simulink model "planmodel2023b"  (R2023b)
settings: Solver=ode4  StartTime=0.0  StopTime=50  FixedStep=0.001  RelTol=1e-3
values from neighbouring files (symbols this model uses):
  a0 = 340.294    [basedata.m]    (also in basedata.mat; control_design.mat; landing_init.m; landing_plan.mat)
  b_ref = 2.0    (= 2)    [basedata.m]    (also in basedata.mat; control_design.mat; landing_init.m; landing_plan.mat)
  c_gear = [0.8e4, 1.4e4, 1.4e4]    [basedata.m]    (also in basedata.mat = [8000 14000 14000]; control_design.mat = [8000 14000 14000]; landing_init.m; landing_plan.mat = [8000 14000 14000])
  c_lat = [1.4e4, 2.2e4, 2.2e4]    [basedata.m]    (also in basedata.mat = [14000 22000 22000]; control_design.mat = [14000 22000 22000]; landing_init.m; landing_plan.mat = [14000 22000 22000])
  c_ref = 0.9    [basedata.m]    (also in basedata.mat; control_design.mat; landing_init.m; landing_plan.mat)
  c_roll = [0.020, 0.018, 0.018]    [basedata.m]    (also in basedata.mat = [0.02 0.018 0.018]; control_design.mat = [0.02 0.018 0.018]; landing_init.m; landing_plan.mat = [0.02 0.018 0.018])
  CD0 = 0.045    [basedata.m]    (also in basedata.mat; canshujisuan.m; control_design.mat; landing_init.m)
  CL0 = 0.083    [basedata.m]    (also in basedata.mat; control_design.mat; landing_init.m; landing_plan.mat)
  CLa = 3.80    (= 3.8)    [basedata.m]    (also in basedata.mat; canshujisuan.m = 2.5; control_design.mat; landing_init.m)
  Clb = -0.08    [basedata.m]    (also in basedata.mat; control_design.mat; landing_init.m; landing_plan.mat)
  Clda = -0.20    (= -0.2)    [basedata.m]    (also in basedata.mat; control_design.mat; landing_init.m; landing_plan.mat)
  CLde = 0.28    [basedata.m]    (also in basedata.mat; control_design.mat; landing_init.m; landing_plan.mat)
  Clp = -0.70    (= -0.7)    [basedata.m]    (also in basedata.mat; control_design.mat; landing_init.m; landing_plan.mat)
  CLq = 4.50    (= 4.5)    [basedata.m]    (also in basedata.mat; canshujisuan.m = 3; control_design.mat; landing_init.m)
  Clr = 0.08    [basedata.m]    (also in basedata.mat; control_design.mat; landing_init.m; landing_plan.mat)
  Cm0 = 0.060    (= 0.06)    [basedata.m]    (also in basedata.mat; control_design.mat; landing_init.m; landing_plan.mat)
  Cma = -0.80    (= -0.8)    [basedata.m]    (also in basedata.mat; control_design.mat; landing_init.m; landing_plan.mat)
  Cmde = -0.90    (= -0.9)    [basedata.m]    (also in basedata.mat; control_design.mat; landing_init.m; landing_plan.mat)
  Cmq = -18.0    (= -18)    [basedata.m]    (also in basedata.mat; control_design.mat; landing_init.m; landing_plan.mat)
  Cnb = 0.25    [basedata.m]    (also in basedata.mat; control_design.mat; landing_init.m; landing_plan.mat)
  Cndr = -0.15    [basedata.m]    (also in basedata.mat; control_design.mat; landing_init.m; landing_plan.mat)
  Cnp = -0.04    [basedata.m]    (also in basedata.mat; control_design.mat; landing_init.m; landing_plan.mat)
  Cnr = -0.45    [basedata.m]    (also in basedata.mat; control_design.mat; landing_init.m; landing_plan.mat)
  CSb = -0.70    (= -0.7)    [basedata.m]    (also in basedata.mat; control_design.mat; landing_init.m; landing_plan.mat)
  CSdr = 0.18    [basedata.m]    (also in basedata.mat; control_design.mat; landing_init.m; landing_plan.mat)
  CSr = 0.12    [basedata.m]    (also in basedata.mat; control_design.mat; landing_init.m; landing_plan.mat)
  D = 0.5 * rho0 * V^2 * S_ref * CD_current    [canshujisuan.m]
  D0 = 1400    [basedata.m]    (also in basedata.mat; control_design.mat = 800; landing.m; landing_init.m)
  da_max = 25    [basedata.m]    (also in basedata.mat; control_design.mat; landing_init.m; landing_plan.mat)
  da_min = -da_max    (= -25)    [basedata.m]    (also in basedata.mat; control_design.mat; landing_init.m; landing_plan.mat)
  de_max = 25    [basedata.m]    (also in basedata.mat; control_design.mat; landing_init.m; landing_plan.mat)
  de_min = -de_max    (= -25)    [basedata.m]    (also in basedata.mat; control_design.mat; landing_init.m; landing_plan.mat)
  DH = pi / 180    (= 0.0174532925199)    [basedata.m]    (also in basedata.mat; control_design.mat; landing_init.m; landing_plan.mat)
  dr_max = 25    [basedata.m]    (also in basedata.mat; control_design.mat; landing_init.m; landing_plan.mat)
  dr_min = -dr_max    (= -25)    [basedata.m]    (also in basedata.mat; control_design.mat; landing_init.m; landing_plan.mat)
  g = 9.80665    [basedata.m]    (also in basedata.mat; canshujisuan.m; control_design.mat; landing_init.m)
  gamma0 = 0.0    (= 0)    [plan.m]    (also in plan.mat)
  ground_y = 0.0    (= 0)    [plan.m]    (also in plan.mat)
  HD = 180 / pi    (= 57.2957795131)    [basedata.m]    (also in basedata.mat; control_design.mat; landing_init.m; landing_plan.mat)
  Ixx = 120.0    (= 120)    [basedata.m]    (also in basedata.mat; control_design.mat; landing_init.m; landing_plan.mat)
  Iyy = 480.0    (= 480)    [basedata.m]    (also in basedata.mat; control_design.mat; landing_init.m; landing_plan.mat)
  Izz = 520.0    (= 520)    [basedata.m]    (also in basedata.mat; control_design.mat; landing_init.m; landing_plan.mat)
  K = 0.12    [basedata.m]    (also in basedata.mat; canshujisuan.m = 0.08; control_design.mat; landing_init.m)
  K_alpha = 7.5375    [basedata.mat]    (also in control_design.m = (((wd_pitch^2)-a24))/(2*kesi_pitch*wd_pitch); control_design.mat; controller.m = 9.375; landingplan.mat)
  k_gear = [1.0e5, 3.0e5, 3.0e5]    [basedata.m]    (also in basedata.mat = [100000 300000 300000]; control_design.mat = [100000 300000 300000]; landing_init.m; landing_plan.mat = [100000 300000 300000])
  k_theta0 = 0.0    (= 0)    [plan.m]    (also in plan.mat)
  Kn_pitch = -0.120095403309    [basedata.mat]    (also in control_design.m = -(2.2*g*(wd_pitch)^2)/(Tr*(((wd_pitch)^2)-a24)*V_control*a34; control_design.mat; controller.m = (2.2*wd^2*g)/(Tr*(wd^2-a24)*V_test*a34); landingplan.mat)
  Kw_pitch = -0.483749055178    [basedata.mat]    (also in control_design.m = -2*kesi_pitch*wd_pitch/a25; control_design.mat; controller.m = -(2*zeta*wd) / a25; landingplan.mat)
  m = 600.0    (= 600)    [basedata.m]    (also in basedata.mat; canshujisuan.m; control_design.mat; landing_init.m)
  mu_brake = [0.0, 0.55, 0.55]    [basedata.m]    (also in basedata.mat = [0 0.55 0.55]; control_design.mat = [0 0.55 0.55]; landing_init.m; landing_plan.mat = [0 0.55 0.55])
  omigax0 = 0    [plan.m]    (also in plan.mat)
  omigay0 = 0    [plan.m]    (also in plan.mat)
  omigaz0 = 0    [plan.m]    (also in plan.mat)
  psi0 = 0    [control_design.mat]    (also in landing.m; landing_init.m; landing_init.mat; landing_plan.mat)
  r_left_b = r_gear_b(:,2)    [basedata.m]    (also in basedata.mat = [-0.333333333333 -0.8 0.65]; control_design.mat = [-0.333333333333 -0.8 0.65]; landing_init.m; landing_plan.mat = [-0.333333333333 -0.8 0.65])
  r_nose_b = r_gear_b(:,1)    [basedata.m]    (also in basedata.mat = [2 0 0.65]; control_design.mat = [2 0 0.65]; landing_init.m; landing_plan.mat = [2 0 0.65])
  r_right_b = r_gear_b(:,3)    [basedata.m]    (also in basedata.mat = [-0.333333333333 0.8 0.65]; control_design.mat = [-0.333333333333 0.8 0.65]; landing_init.m; landing_plan.mat = [-0.333333333333 0.8 0.65])
  rho0 = 1.225    [basedata.m]    (also in basedata.mat; canshujisuan.m; control_design.mat; landing_init.m)
  S_ref = 1.2    [basedata.m]    (also in basedata.mat; canshujisuan.m; control_design.mat; landing_init.m)
  v_eps = 0.20    (= 0.2)    [basedata.m]    (also in basedata.mat; control_design.mat; landing_init.m; landing_plan.mat)
  V_min = 3    [control_design.mat]    (also in landing.m; landing_init.m; landing_plan.mat; landingplan.mat)
  Vx0_b = 0.0    (= 0)    [plan.m]    (also in plan.mat)
  Vy0_b = 0.0    (= 0)    [plan.m]    (also in plan.mat)
  Vz0_b = 0.0    (= 0)    [plan.m]    (also in plan.mat)
  wheel_radius = 0.18    [basedata.m]    (also in basedata.mat; control_design.mat; landing_init.m; landing_plan.mat)
  WOW_on = 0.000    (= 0)    [basedata.m]    (also in basedata.mat; control_design.mat; landing_init.m; landing_plan.mat)
  Xg0 = 0    [control_design.mat]    (also in landing.m = -12000; landing_init.m = -12000; landing_init.mat = -8000; landing_plan.mat = -12000)
  Yg0 = 3    [control_design.mat]    (also in landing.m = 0; landing_init.m = 0; landing_init.mat = 0; landing_plan.mat = 0)
  Zg0 = ground_z - wheel_radius - r_gear_b(3,1) + static_deflection    [basedata.m]    (also in basedata.mat = -0.8215943; control_design.mat = -0.8215943; landing.m = -1000; landing_init.m = -1000)
libraries: matrix_library x18, slpidlib x1
(part 3 of 3)

== matlab function planmodel2023b/control/MATLAB Function ==
  settings: updateMethod=DISCRETE
  data: Vx input; theta_cmd output; no_contact input; t input; theta_actual input
function theta_cmd = fcn(Vx, no_contact, t, theta_actual)
% 起飞抬前轮俯仰角指令生成
% Vx:           机体系前向速度 (m/s)
% no_contact:   无轮接地信号, 1=空中, 0=地面
% t:            仿真时间 (s), 接 Digital Clock
% theta_actual: 飞机当前的实际俯仰角 (rad), 用于离地无缝切换

persistent t_rotation
persistent theta_takeoff_hold

if isempty(t_rotation)
    t_rotation = inf;
end
if isempty(theta_takeoff_hold)
    theta_takeoff_hold = 0;
end

%% --- 参数配置（根据实际机型调整） ---
VR = 50;                      % m/s, 抬轮速度 
theta_target = 12 * pi/180;   % rad, 目标俯仰角锁定在 10°
rotation_rate = 4 * pi/180;   % rad/s, 抬轮角速率设定为 3°/s，平稳抬头

%% --- 状态机控制逻辑 ---
if no_contact > 0.5
    % 【空中阶段】
    % 刚离地瞬间，记录下离地时的实际姿态，防止指令断崖式下掉
    if theta_takeoff_hold == 0
        theta_takeoff_hold = theta_actual; 
    end
    
    % 在这里，theta_cmd 应该输出离地锁定的姿态，或者直接交给空中的俯仰回路
    % 绝对不能直接置 0！
    theta_cmd = theta_takeoff_hold; 
    
    % 重置滑跑计时器
    t_rotation = inf;

elseif Vx >= VR
    % 【抬轮阶段】
    if isinf(t_rotation)
        t_rotation = t;       % 记录开始抬轮的绝对时间
    end
    
    % 按照设定的速率（3°/s）线性增加俯仰角指令
    theta_cmd = rotation_rate * (t - t_rotation);
    
    % 达到目标角度（10°）后进行限幅切顶
    if theta_cmd > theta_target
        theta_cmd = theta_target;
    end
    
    % 尚未离地，清空离地保持值
    theta_takeoff_hold = 0;

else
    % 【地面加速滑跑阶段】
    % 保持前轮三点接地姿态（通常为 0° 或略微带一点下俯角压前轮，视安装角而定）
    theta_cmd = -4*pi/180; 
    t_rotation = inf;
    theta_takeoff_hold = 0;
end% 在你的状态机逻辑中添加：

end

== matlab function planmodel2023b/6DOF-MODEL/动力学/体系旋转角速度/MATLAB Function ==
  data: alpha input; R_wind_b output; beta input
 function R_wind_b = wind2body(alpha, beta)
T1 = [cos(beta), 0, -sin(beta);
       0, 1, 0;
       sin(beta), 0, cos(beta)];
T2 = [cos(alpha), sin(alpha), 0;
       -sin(alpha), cos(alpha), 0;
       0, 0, 1];
R_wind_b = T2*T1;

== matlab function planmodel2023b/6DOF-MODEL/动力学/Subsystem3/MATLAB Function1 ==
  data: gamma input; R_gb output; theta input; psi input
function R_gb = ground2body(gamma, theta, psi)
    T1=[cos(psi), 0 ,-sin(psi);...
          0     , 1 ,    0   ;...
        sin(psi), 0 ,cos(psi);];%绕y偏航
    T2=[cos(theta),sin(theta),0;...
        -sin(theta),cos(theta),0;...
          0        , 0 ,       1;];%绕z俯仰角
    T3=[1,0,0;...
        0,cos(gamma),sin(gamma);...
        0,-sin(gamma),cos(gamma);];%绕x滚转角

   R_gb=T3*T2*T1;

== matlab function planmodel2023b/6DOF-MODEL/动力学/起落架模型/起落架三轮质心在地系下位置/MATLAB Function1 ==
  data: gamma input; R_gb output; theta input; psi input
function R_gb = ground2body(gamma, theta, psi)
    T1=[cos(psi), 0 ,-sin(psi);...
          0     , 1 ,    0   ;...
        sin(psi), 0 ,cos(psi);];%绕y偏航
    T2=[cos(theta),sin(theta),0;...
        -sin(theta),cos(theta),0;...
          0        , 0 ,       1;];%绕z俯仰角
    T3=[1,0,0;...
        0,cos(gamma),sin(gamma);...
        0,-sin(gamma),cos(gamma);];%绕x滚转角

   R_gb=T3*T2*T1;

== matlab function planmodel2023b/6DOF-MODEL/动力学/height/MATLAB Function2 ==
  data: gamma input; R_gb output; theta input; psi input
function R_gb = ground2body(gamma, theta, psi)
    T1=[cos(psi), 0 ,-sin(psi);...
          0     , 1 ,    0   ;...
        sin(psi), 0 ,cos(psi);];%绕y偏航
    T2=[cos(theta),sin(theta),0;...
        -sin(theta),cos(theta),0;...
          0        , 0 ,       1;];%绕z俯仰角
    T3=[1,0,0;...
        0,cos(gamma),sin(gamma);...
        0,-sin(gamma),cos(gamma);];%绕x滚转角

   R_gb=T3*T2*T1;

== matlab function planmodel2023b/6DOF-MODEL/动力学/v在体系下的分量/MATLAB Function ==
  data: alpha input; R_wind_b output; beta input
 function R_wind_b = wind2body(alpha, beta)
T1 = [cos(beta), 0, -sin(beta);
       0, 1, 0;
       sin(beta), 0, cos(beta)];
T2 = [cos(alpha), sin(alpha), 0;
       -sin(alpha), cos(alpha), 0;
       0, 0, 1];
R_wind_b = T2*T1;

== matlab function planmodel2023b/6DOF-MODEL/动力学/v在体系下的分量/MATLAB Function1 ==
  data: gamma input; R_gb output; theta input; psi input
function R_gb = ground2body(gamma, theta, psi)
    T1=[cos(psi), 0 ,-sin(psi);...
          0     , 1 ,    0   ;...
        sin(psi), 0 ,cos(psi);];%绕y偏航
    T2=[cos(theta),sin(theta),0;...
        -sin(theta),cos(theta),0;...
          0        , 0 ,       1;];%绕z俯仰角
    T3=[1,0,0;...
        0,cos(gamma),sin(gamma);...
        0,-sin(gamma),cos(gamma);];%绕x滚转角

   R_gb=T3*T2*T1;

== matlab function planmodel2023b/6DOF-MODEL/动力学/起落架模型/法向支反力/MATLAB Function1 ==
  data: gamma input; R_gb output; theta input; psi input
function R_gb = ground2body(gamma, theta, psi)
    T1=[cos(psi), 0 ,-sin(psi);...
          0     , 1 ,    0   ;...
        sin(psi), 0 ,cos(psi);];%绕y偏航
    T2=[cos(theta),sin(theta),0;...
        -sin(theta),cos(theta),0;...
          0        , 0 ,       1;];%绕z俯仰角
    T3=[1,0,0;...
        0,cos(gamma),sin(gamma);...
        0,-sin(gamma),cos(gamma);];%绕x滚转角

   R_gb=T3*T2*T1;

== matlab function planmodel2023b/6DOF-MODEL/动力学/起落架模型/纵向力/Subsystem/MATLAB Function1 ==
  data: gamma input; R_gb output; theta input; psi input
function R_gb = ground2body(gamma, theta, psi)
    T1=[cos(psi), 0 ,-sin(psi);...
          0     , 1 ,    0   ;...
        sin(psi), 0 ,cos(psi);];%绕y偏航
    T2=[cos(theta),sin(theta),0;...
        -sin(theta),cos(theta),0;...
          0        , 0 ,       1;];%绕z俯仰角
    T3=[1,0,0;...
        0,cos(gamma),sin(gamma);...
        0,-sin(gamma),cos(gamma);];%绕x滚转角

   R_gb=T3*T2*T1;

== matlab function planmodel2023b/6DOF-MODEL/动力学/起落架模型/纵向力/Subsystem/前轮滚动方向向量 ==
  data: Cbg input; eg_long output; eb_long input
function eg_long= project_long(Cbg,eb_long)

e_y=[0;1;0];
P_g=eye(3)-e_y*e_y';
eg_long=P_g*Cbg*eb_long;
eg_long=eg_long/norm(eg_long);

== matlab function planmodel2023b/6DOF-MODEL/动力学/起落架模型/纵向力/Subsystem/主轮滚动方向向量 ==
  data: Cbg input; eg_long output; eb_long input
function eg_long= project_long(Cbg,eb_long)


e_y=[0;1;0];
P_g=eye(3)-e_y*e_y';

eg_long=P_g*Cbg*eb_long;
eg_long=eg_long/norm(eg_long);
